simulink model "gyroSystem"  (R2018a)
settings: Solver=VariableStepAuto  StartTime=0.0  StopTime=10.0  RelTol=1e-3
libraries: dspspect3 x2
settings Model: Creator=Dario Quintero  LastModifiedBy=Dario Quintero
settings DataIOCC: ReturnWorkspaceOutputs=on
settings SFSimCC: SimUseLocalCustomCode=on
settings RTWCC: RTWUseLocalCustomCode=on

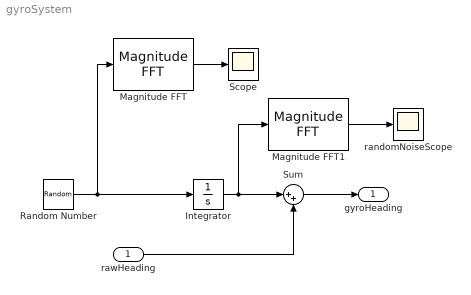
== system gyroSystem ==
  rawHeading : Inport
  Integrator : Integrator
  Magnitude FFT : dspspect3/Magnitude FFT  mag_or_magsq=Magnitude  FFTImplementation=Auto  fftLenInherit=off  fftsize=256  WrapInput=on
      settings: SourceProductName=DSP System Toolbox  SourceProductBaseCode=DS
  Magnitude FFT1 : dspspect3/Magnitude FFT  mag_or_magsq=Magnitude  FFTImplementation=Auto  fftLenInherit=off  fftsize=256  WrapInput=on
      settings: SourceProductName=DSP System Toolbox  SourceProductBaseCode=DS
  Random Number : RandomNumber  Mean=0.02  Variance=0.01  SampleTime=0.1
  Scope : Scope
  Sum : Sum  Inputs=|++
  randomNoiseScope : Scope
  gyroHeading : Outport
  wires:
  Random Number/1 -> Magnitude FFT/1, Integrator/1
  Integrator/1 -> Sum/1, Magnitude FFT1/1
  rawHeading/1 -> Sum/2
  Sum/1 -> gyroHeading/1
  Magnitude FFT/1 -> Scope/1
  Magnitude FFT1/1 -> randomNoiseScope/1
